simulink model "DAS"  (R2012b)
settings: Solver=FixedStepDiscrete  StartTime=0.0  StopTime=inf  FixedStep=0.1  RelTol=1e-3
PreLoadFcn:
  | if exist('tl_preloadfcn','file'), tl_preloadfcn(gcs,101); end
PostLoadFcn:
  | if exist('tl_postloadfcn','file'), tl_postloadfcn(gcs,101); end
InitFcn:
  | if exist('tlds_init','file'), tlds_init(gcs); end
StartFcn:
  | if exist('tlds_start','file'), tlds_start(gcs); end
StopFcn:
  | if exist('tlds_stop','file'), tlds_stop(gcs); end
undefined symbols (not defined in the file): A, B, C, Dd, DEMO_FAS_Accusti_Threshold_Time, DEMO_FAS_BrakeBooster_Threshold, DEMO_FAS_CC_DELTA, DEMO_FAS_CC_Lvl2_Round, DEMO_FAS_CC_Min_Value, DEMO_FAS_Distance_Treshold_Far, DEMO_FAS_Distance_Treshold_Med, DEMO_FAS_Distance_Treshold_Near, DEMO_FAS_Distronic, DEMO_FAS_Emerg_Brake_Force1, DEMO_FAS_Emerg_Brake_Force2, DEMO_FAS_Emerg_Brake_Time1, DEMO_FAS_Emerg_Brake_Time2, DEMO_FAS_EmergencyBrake, DEMO_FAS_FollowToStop, DEMO_FAS_Limiter, DEMO_FAS_Limiter_DELTA, DEMO_FAS_Neg_Max_ms, DEMO_FAS_Opti_Threshold_Time, DEMO_FAS_Repeater, DEMO_FAS_Repeater_Time, DEMO_FAS_Signdetection, DEMO_FAS_Tempomat
(part 6 of 11)

== system DAS/DEMO_FAS/DEMO_FAS/Subsystem/DEMO_FAS/DEMO_FAS_Funktion/Limiter/Limiter_Function/Limiter_SetValue ==
  LeverUp_stat : Inport
  LeverDown_stat : Inport  Port=2
  Enable : EnablePort
  Constant1 : Constant  Value=0  mask(TL_Constant){data={'date',735340.38498962962}}
      settings: CopyFcn=if exist('tl_reset_reviewflag') == 2, tl_reset_reviewflag(gcbh); end  DeleteFcn=if exist('delete_tlblock','file')==2,delete_tlblock(gcbh);end  NameChangeFcn=if exist('rename_tlblock','file')==2,rename_tlblock(gcbh);end  OpenFcn=if exist('tl_open_blockdlg','file')==2,tl_open_blockdlg(gcbh);else,open_system(gcbh,'parameter');end
      mask Help: eval(['if exist(''tl_online_help'',''file'') == 2, tl_online_help(''Topic'',''TL_Constant''),else, web([''jar:file:///'',matlabroot,''/help/toolbox/simulink/help.jar!/slref/' lower(get_param(gcbh,'Blocktype')) '.html''], ''-helpbrowser''),end'])
      mask Display: plot([-0.05, 1.05, NaN, -0.05, 1.05],[.01, .01, NaN, .99, .99])
  Constant3 : Constant  Value=0  mask(TL_Constant){data={'date',735340.38498962962}}
      settings: CopyFcn=if exist('tl_reset_reviewflag') == 2, tl_reset_reviewflag(gcbh); end  DeleteFcn=if exist('delete_tlblock','file')==2,delete_tlblock(gcbh);end  NameChangeFcn=if exist('rename_tlblock','file')==2,rename_tlblock(gcbh);end  OpenFcn=if exist('tl_open_blockdlg','file')==2,tl_open_blockdlg(gcbh);else,open_system(gcbh,'parameter');end
      mask Help: eval(['if exist(''tl_online_help'',''file'') == 2, tl_online_help(''Topic'',''TL_Constant''),else, web([''jar:file:///'',matlabroot,''/help/toolbox/simulink/help.jar!/slref/' lower(get_param(gcbh,'Blocktype')) '.html''], ''-helpbrowser''),end'])
      mask Display: plot([-0.05, 1.05, NaN, -0.05, 1.05],[.01, .01, NaN, .99, .99])
  Data Store Read1 : DataStoreRead  Description=|  DataStoreName=DEMO_FAS_V_LimiterSetValue  mask(TL_DataStoreRead){data={'logdata',{'plotchannels',[]},'date',735342.5274069329}}
      | Data Store Read block of dSPACE TargetLink.
      | Use this block to specify inputs from global variables within the production code application.
      settings: DeleteFcn=if exist('delete_tlblock','file')==2,delete_tlblock(gcbh);end  NameChangeFcn=if exist('rename_tlblock','file')==2,rename_tlblock(gcbh);end  OpenFcn=if exist('tl_open_blockdlg','file')==2,tl_open_blockdlg(gcbh);else,open_system(gcbh,'parameter');end
      mask Help: eval(['if exist(''tl_online_help'',''file'') == 2, tl_online_help(''Topic'',''TL_DataStoreRead''),else, web([''jar:file:///'',matlabroot,''/help/toolbox/simulink/help.jar!/slref/' lower(get_param(gcbh,'Blocktype')) '.html''], ''-helpbrowser''),end'])
      mask Display: plot([-0.05, 1.05, NaN, -0.05, 1.05],[.01, .01, NaN, .99, .99])
  RelOp1 : RelationalOperator  Description=|  Operator=>  mask(TL_RelationalOperator){data={'logdata',{'plotchannels',[]},'date',735370.55844204861}}
      | Relational operator block of dSPACE TargetLink.
      | 
      | This block performs a relational operation on its two inputs u1 and u2 and produces output according to the following table.
      | If the result is TRUE, the output is 1; if FALSE, it is 0.
      | 
      | Operator   Output
      |  ==        TRUE if u1 is equal to u2
      |  !=        TRUE if u1 is not equal to u2
      |  <         TRUE if u1 is less than u2
      |  <=        TRUE if u1 is less than or equal to u2
      |  >=        TRUE if u1 is greater than or equal to u2
      |  >         TRUE if u1 is greater than u2
      settings: DeleteFcn=if exist('delete_tlblock','file')==2,delete_tlblock(gcbh);end  NameChangeFcn=if exist('rename_tlblock','file')==2,rename_tlblock(gcbh);end  OpenFcn=if exist('tl_open_blockdlg','file')==2,tl_open_blockdlg(gcbh);else,open_system(gcbh,'parameter');end
      mask Help: eval(['if exist(''tl_online_help'',''file'') == 2, tl_online_help(''Topic'',''TL_RelationalOperator''),else, web([''jar:file:///'',matlabroot,''/help/toolbox/simulink/help.jar!/slref/' lower(get_param(gcbh,'Blocktype')) '.html''], ''-helpbrowser''),end'])
      mask Display: plot([-0.05, 1.05, NaN, -0.05, 1.05],[.01, .01, NaN, .99, .99])
  RelOp3 : RelationalOperator  Description=|  Operator=>  mask(TL_RelationalOperator){data={'logdata',{'plotchannels',[]},'date',735370.55844204861}}
      | Relational operator block of dSPACE TargetLink.
      | 
      | This block performs a relational operation on its two inputs u1 and u2 and produces output according to the following table.
      | If the result is TRUE, the output is 1; if FALSE, it is 0.
      | 
      | Operator   Output
      |  ==        TRUE if u1 is equal to u2
      |  !=        TRUE if u1 is not equal to u2
      |  <         TRUE if u1 is less than u2
      |  <=        TRUE if u1 is less than or equal to u2
      |  >=        TRUE if u1 is greater than or equal to u2
      |  >         TRUE if u1 is greater than u2
      settings: DeleteFcn=if exist('delete_tlblock','file')==2,delete_tlblock(gcbh);end  NameChangeFcn=if exist('rename_tlblock','file')==2,rename_tlblock(gcbh);end  OpenFcn=if exist('tl_open_blockdlg','file')==2,tl_open_blockdlg(gcbh);else,open_system(gcbh,'parameter');end
      mask Help: eval(['if exist(''tl_online_help'',''file'') == 2, tl_online_help(''Topic'',''TL_RelationalOperator''),else, web([''jar:file:///'',matlabroot,''/help/toolbox/simulink/help.jar!/slref/' lower(get_param(gcbh,'Blocktype')) '.html''], ''-helpbrowser''),end'])
      mask Display: plot([-0.05, 1.05, NaN, -0.05, 1.05],[.01, .01, NaN, .99, .99])
  VERSION_INFO : Subsystem  mask(VERSION_INFO_BLOCK){versinfo_data=struct('modname','DEMO_FAS/DEMO_FAS_Funktion/Limiter/Limiter_Function/Limiter_SetValue','version','1.1.1','date','18-Apr-2013','author','YVEDUHR','modtype',3,'variant',0,'remark',{{'~'}},'copyright',['Daimler AG'],'SGMLdescr','','prefix','','pfx_act',0,'ntselect',3,'asize',0), versinfo_string=Model: DEMO_FAS/DEMO_FAS_Funktion/Limiter/Limiter_Function/Limiter_SetValue\nVersion: 1.1.1\nDate: 18-Apr-2013\nAuthor: YVEDUHR\nModule: INTERNAL\n\nAll copyrights by Daimler AG}
      mask prompts: versinfo_data "Mask Parameter 1"; versinfo_string "Mask Parameter 2"
      mask help:
      | This is a Version Info Subsystem (empty)
      | All version Information is stored in Parameter "versinfo_data" and displayed
      settings: OpenFcn=edit_subsys_info('init')
      mask Display: disp(versinfo_string);
  V_LimSetValueMinus : Subsystem  TreatAsAtomicUnit=on
  V_LimSetValuePlus : Subsystem  TreatAsAtomicUnit=on
  wires:
  LeverDown_stat/1 -> RelOp1/1
  LeverUp_stat/1 -> RelOp3/1
  Data Store Read1/1 -> V_LimSetValuePlus/1(V_LimiterSetValue), V_LimSetValueMinus/1(V_LimiterSetValue)  "V_LimiterSetValue"
  RelOp3/1 -> V_LimSetValuePlus/Trigger
  Constant3/1 -> RelOp3/2
  Constant1/1 -> RelOp1/2
  RelOp1/1 -> V_LimSetValueMinus/Trigger

== system DAS/DEMO_FAS/DEMO_FAS/Subsystem/DEMO_FAS/DEMO_FAS_Funktion/Limiter/Limiter_Function/Limiter_StartUpSetValue ==
  Trigger : TriggerPort
  Constant : Constant  Value=300  mask(TL_Constant){data={'date',735343.44782005786}}
      settings: CopyFcn=if exist('tl_reset_reviewflag') == 2, tl_reset_reviewflag(gcbh); end  DeleteFcn=if exist('delete_tlblock','file')==2,delete_tlblock(gcbh);end  NameChangeFcn=if exist('rename_tlblock','file')==2,rename_tlblock(gcbh);end  OpenFcn=if exist('tl_open_blockdlg','file')==2,tl_open_blockdlg(gcbh);else,open_system(gcbh,'parameter');end
      mask Help: eval(['if exist(''tl_online_help'',''file'') == 2, tl_online_help(''Topic'',''TL_Constant''),else, web([''jar:file:///'',matlabroot,''/help/toolbox/simulink/help.jar!/slref/' lower(get_param(gcbh,'Blocktype')) '.html''], ''-helpbrowser''),end'])
      mask Display: plot([-0.05, 1.05, NaN, -0.05, 1.05],[.01, .01, NaN, .99, .99])
  Data Store Write : DataStoreWrite  Description=|  DataStoreName=DEMO_FAS_V_CCSetValue  mask(TL_DataStoreWrite){data={'date',735342.52876391204}}
      | Data Store Write block of dSPACE TargetLink.
      | Use this block to specify outputs to global variables within the production code application.
      settings: DeleteFcn=if exist('delete_tlblock','file')==2,delete_tlblock(gcbh);end  NameChangeFcn=if exist('rename_tlblock','file')==2,rename_tlblock(gcbh);end  OpenFcn=if exist('tl_open_blockdlg','file')==2,tl_open_blockdlg(gcbh);else,open_system(gcbh,'parameter');end
      mask Help: eval(['if exist(''tl_online_help'',''file'') == 2, tl_online_help(''Topic'',''TL_DataStoreWrite''),else, web([''jar:file:///'',matlabroot,''/help/toolbox/simulink/help.jar!/slref/' lower(get_param(gcbh,'Blocktype')) '.html''], ''-helpbrowser''),end'])
      mask Display: plot([-0.05, 1.05, NaN, -0.05, 1.05],[.01, .01, NaN, .99, .99])
  VERSION_INFO : Subsystem  mask(VERSION_INFO_BLOCK){versinfo_data=struct('modname','DEMO_FAS/DEMO_FAS_Funktion/Limiter/Limiter_Function/Limiter_StartUpSetValue','version','1.1.1','date','18-Apr-2013','author','YVEDUHR','modtype',3,'variant',0,'remark',{{'~'}},'copyright',['Daimler AG'],'SGMLdescr','','prefix','','pfx_act',0,'ntselect',3,'asize',0), versinfo_string=Model: DEMO_FAS/DEMO_FAS_Funktion/Limiter/Limiter_Function/Limiter_StartUpSetValue\nVersion: 1.1.1\nDate: 18-Apr-2013\nAuthor: YVEDUHR\nModule: INTERNAL\n\nAll copyrights by Daimler AG}
      mask prompts: versinfo_data "Mask Parameter 1"; versinfo_string "Mask Parameter 2"
      mask help:
      | This is a Version Info Subsystem (empty)
      | All version Information is stored in Parameter "versinfo_data" and displayed
      settings: OpenFcn=edit_subsys_info('init')
      mask Display: disp(versinfo_string);
  wires:
  Constant/1 -> Data Store Write/1

== system DAS/DEMO_FAS/DEMO_FAS/Subsystem/DEMO_FAS/DEMO_FAS_Funktion/Limiter/Limiter_Function/SysInit ==
  Memory_Init : UnitDelay  Description=|  InitialCondition=1  SampleTime=dT  mask(TL_UnitDelay){data={'logdata',{'plotchannels',[]},'output',{'type','Bool'},'state',{'type','Bool'},'date',734383.73415}}
      | Unit Delay block of dSPACE TargetLink.
      | 
      | Output signal is equal to the input signal of the last sample step:
      | 
      |         y(k) = u(k-1).
      | 
      | In the 1st sampling step, the output signal is initialized with 'initial condition':
      | 
      |         y(0) = initial condition
      settings: CopyFcn=if exist('tl_reset_reviewflag') == 2, tl_reset_reviewflag(gcbh); end  DeleteFcn=if exist('delete_tlblock','file')==2,delete_tlblock(gcbh);end  NameChangeFcn=if exist('rename_tlblock','file')==2,rename_tlblock(gcbh);end  OpenFcn=if exist('tl_open_blockdlg','file')==2,tl_open_blockdlg(gcbh);else,open_system(gcbh,'parameter');end
      mask Help: eval(['if exist(''tl_online_help'',''file'') == 2, tl_online_help(''Topic'',''TL_UnitDelay''),else, web([''jar:file:///'',matlabroot,''/help/toolbox/simulink/help.jar!/slref/' lower(get_param(gcbh,'Blocktype')) '.html''], ''-helpbrowser''),end'])
      mask Display: plot([-0.05, 1.05, NaN, -0.05, 1.05],[.01, .01, NaN, .99, .99])
  Zero_Init : Constant  Description=|  Value=0  SampleTime=dT  mask(TL_Constant){data={'date',734383.73414928245}}
      | Constant block of dSPACE TargetLink.
      | 
      | Output signal keeps the given constant value.
      settings: DeleteFcn=if exist('delete_tlblock','file')==2,delete_tlblock(gcbh);end  NameChangeFcn=if exist('rename_tlblock','file')==2,rename_tlblock(gcbh);end  OpenFcn=if exist('tl_open_blockdlg','file')==2,tl_open_blockdlg(gcbh);else,open_system(gcbh,'parameter');end
      mask Help: eval(['if exist(''tl_online_help'',''file'') == 2, tl_online_help(''Topic'',''TL_Constant''),else, web([''jar:file:///'',matlabroot,''/help/toolbox/simulink/help.jar!/slref/' lower(get_param(gcbh,'Blocktype')) '.html''], ''-helpbrowser''),end'])
      mask Display: plot([-0.05, 1.05, NaN, -0.05, 1.05],[.01, .01, NaN, .99, .99])
  y : Outport
  wires:
  Zero_Init/1 -> Memory_Init/1
  Memory_Init/1 -> y/1

== system DAS/DEMO_FAS/DEMO_FAS/Subsystem/DEMO_FAS/DEMO_FAS_Funktion/Limiter/Limiter_Function/VERSION_INFO ==
  Copyright : Subsystem
      mask help: Copyright
      mask Display: disp('All copyrights by DaimlerChrysler');

== system DAS/DEMO_FAS/DEMO_FAS/Subsystem/DEMO_FAS/DEMO_FAS_Funktion/Limiter/VERSION_INFO/Copyright ==

== system DAS/DEMO_FAS/DEMO_FAS/Subsystem/DEMO_FAS/DEMO_FAS_Funktion/Tempomat/Tempomat_Function/CC_Enabled ==
  CC_active_b : Inport
  V_Vehicle_kmh : Inport  Port=2
  Bus Creator : BusCreator  Inputs=1
  Bus Creator1 : BusCreator  Inputs=1
  Bus Selector : BusSelector  OutputSignals=V_CC_delta_kmh
  If : If  IfExpression=u1
  Merge : Merge  Description=|  mask(TL_Merge){data={'date',735441.37248614582}}
      | Merge block of dSPACE TargetLink.
      | 
      | Use this block instead of Simulink's Merge block if you wish to control how merge variables should be generated.
      settings: CopyFcn=if exist('tl_reset_reviewflag') == 2, tl_reset_reviewflag(gcbh); end  DeleteFcn=if exist('delete_tlblock','file')==2,delete_tlblock(gcbh);end  NameChangeFcn=if exist('rename_tlblock','file')==2,rename_tlblock(gcbh);end  OpenFcn=if exist('tl_open_blockdlg','file')==2,tl_open_blockdlg(gcbh);else,open_system(gcbh,'parameter');end
      mask Help: eval(['if exist(''tl_online_help'',''file'') == 2, tl_online_help(''Topic'',''TL_Merge''),else, web([''jar:file:///'',matlabroot,''/help/toolbox/simulink/help.jar!/slref/' lower(get_param(gcbh,'Blocktype')) '.html''], ''-helpbrowser''),end'])
      mask Display: plot([-0.05, 1.05, NaN, -0.05, 1.05],[.01, .01, NaN, .99, .99])
  Tempomat_Active : Subsystem  TreatAsAtomicUnit=on
  Tempomat_Deactive : Subsystem  TreatAsAtomicUnit=on
  VERSION_INFO : Subsystem  mask(VERSION_INFO_BLOCK){versinfo_data=struct('modname','DEMO_FAS/DEMO_FAS_Funktion/Tempomat/Tempomat_Function/CC_Enabled','version','1.1.1','date','18-Apr-2013','author','YVEDUHR','modtype',3,'variant',0,'remark',{{'~'}},'copyright',['Daimler AG'],'SGMLdescr','','prefix','','pfx_act',0,'ntselect',3,'asize',0), versinfo_string=Model: DEMO_FAS/DEMO_FAS_Funktion/Tempomat/Tempomat_Function/CC_Enabled\nVersion: 1.1.1\nDate: 18-Apr-2013\nAuthor: YVEDUHR\nModule: INTERNAL\n\nAll copyrights by Daimler AG}
      mask prompts: versinfo_data "Mask Parameter 1"; versinfo_string "Mask Parameter 2"
      mask help:
      | This is a Version Info Subsystem (empty)
      | All version Information is stored in Parameter "versinfo_data" and displayed
      settings: OpenFcn=edit_subsys_info('init')
      mask Display: disp(versinfo_string);
  V_CC_delta_kmh : Outport  InitialOutput=0
  wires:
  If/1 -> Tempomat_Active/Action
  V_Vehicle_kmh/1 -> Tempomat_Active/1(V_Vehicle_kmh)
  Tempomat_Active/1(V_CC_delta_kmh) -> Bus Creator/1
  Bus Creator/1 -> Merge/1
  Tempomat_Deactive/1(V_CC_delta_kmh) -> Bus Creator1/1
  Bus Creator1/1 -> Merge/2
  Merge/1 -> Bus Selector/1  "V_CC_delta_kmh"
  Bus Selector/1 -> V_CC_delta_kmh/1  "<V_CC_delta_kmh>"
  CC_active_b/1 -> If/1
  If/2 -> Tempomat_Deactive/Action

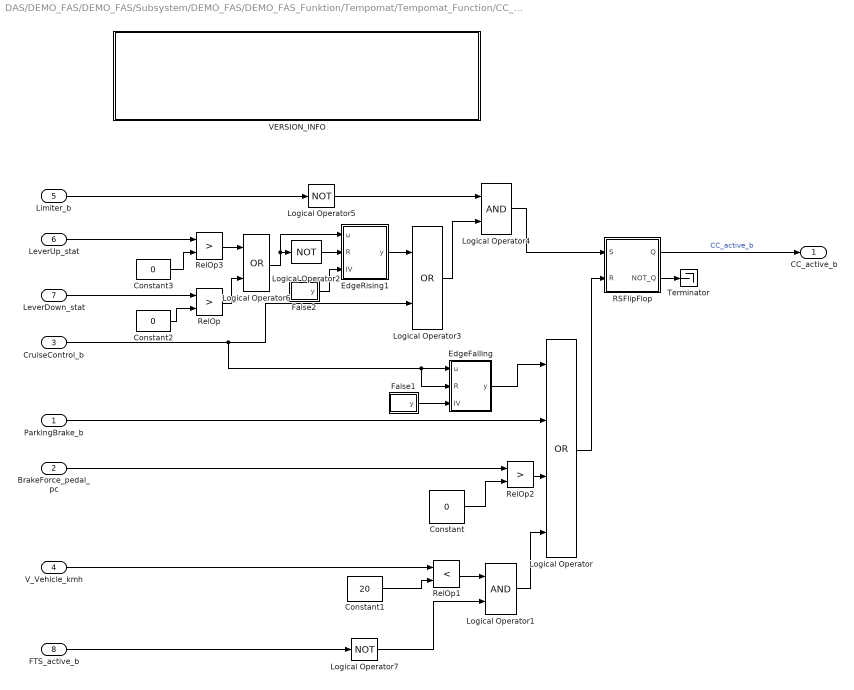
== system DAS/DEMO_FAS/DEMO_FAS/Subsystem/DEMO_FAS/DEMO_FAS_Funktion/Tempomat/Tempomat_Function/CC_On_Off ==
  ParkingBrake_b : Inport
  BrakeForce_pedal_pc : Inport  Port=2
  CruiseControl_b : Inport  Port=3
  V_Vehicle_kmh : Inport  Port=4
  Limiter_b : Inport  Port=5
  LeverUp_stat : Inport  Port=6
  LeverDown_stat : Inport  Port=7
  FTS_active_b : Inport  Port=8
  Constant : Constant  Value=0  mask(TL_Constant){data={'date',735340.38498962962}}
      settings: CopyFcn=if exist('tl_reset_reviewflag') == 2, tl_reset_reviewflag(gcbh); end  DeleteFcn=if exist('delete_tlblock','file')==2,delete_tlblock(gcbh);end  NameChangeFcn=if exist('rename_tlblock','file')==2,rename_tlblock(gcbh);end  OpenFcn=if exist('tl_open_blockdlg','file')==2,tl_open_blockdlg(gcbh);else,open_system(gcbh,'parameter');end
      mask Help: eval(['if exist(''tl_online_help'',''file'') == 2, tl_online_help(''Topic'',''TL_Constant''),else, web([''jar:file:///'',matlabroot,''/help/toolbox/simulink/help.jar!/slref/' lower(get_param(gcbh,'Blocktype')) '.html''], ''-helpbrowser''),end'])
      mask Display: plot([-0.05, 1.05, NaN, -0.05, 1.05],[.01, .01, NaN, .99, .99])
  Constant1 : Constant  Value=20  mask(TL_Constant){data={'date',735343.57031072921}}
      settings: CopyFcn=if exist('tl_reset_reviewflag') == 2, tl_reset_reviewflag(gcbh); end  DeleteFcn=if exist('delete_tlblock','file')==2,delete_tlblock(gcbh);end  NameChangeFcn=if exist('rename_tlblock','file')==2,rename_tlblock(gcbh);end  OpenFcn=if exist('tl_open_blockdlg','file')==2,tl_open_blockdlg(gcbh);else,open_system(gcbh,'parameter');end
      mask Help: eval(['if exist(''tl_online_help'',''file'') == 2, tl_online_help(''Topic'',''TL_Constant''),else, web([''jar:file:///'',matlabroot,''/help/toolbox/simulink/help.jar!/slref/' lower(get_param(gcbh,'Blocktype')) '.html''], ''-helpbrowser''),end'])
      mask Display: plot([-0.05, 1.05, NaN, -0.05, 1.05],[.01, .01, NaN, .99, .99])
  Constant2 : Constant  Value=0  mask(TL_Constant){data={'date',735340.38498962962}}
      settings: CopyFcn=if exist('tl_reset_reviewflag') == 2, tl_reset_reviewflag(gcbh); end  DeleteFcn=if exist('delete_tlblock','file')==2,delete_tlblock(gcbh);end  NameChangeFcn=if exist('rename_tlblock','file')==2,rename_tlblock(gcbh);end  OpenFcn=if exist('tl_open_blockdlg','file')==2,tl_open_blockdlg(gcbh);else,open_system(gcbh,'parameter');end
      mask Help: eval(['if exist(''tl_online_help'',''file'') == 2, tl_online_help(''Topic'',''TL_Constant''),else, web([''jar:file:///'',matlabroot,''/help/toolbox/simulink/help.jar!/slref/' lower(get_param(gcbh,'Blocktype')) '.html''], ''-helpbrowser''),end'])
      mask Display: plot([-0.05, 1.05, NaN, -0.05, 1.05],[.01, .01, NaN, .99, .99])
  Constant3 : Constant  Value=0  mask(TL_Constant){data={'date',735340.38498962962}}
      settings: CopyFcn=if exist('tl_reset_reviewflag') == 2, tl_reset_reviewflag(gcbh); end  DeleteFcn=if exist('delete_tlblock','file')==2,delete_tlblock(gcbh);end  NameChangeFcn=if exist('rename_tlblock','file')==2,rename_tlblock(gcbh);end  OpenFcn=if exist('tl_open_blockdlg','file')==2,tl_open_blockdlg(gcbh);else,open_system(gcbh,'parameter');end
      mask Help: eval(['if exist(''tl_online_help'',''file'') == 2, tl_online_help(''Topic'',''TL_Constant''),else, web([''jar:file:///'',matlabroot,''/help/toolbox/simulink/help.jar!/slref/' lower(get_param(gcbh,'Blocktype')) '.html''], ''-helpbrowser''),end'])
      mask Display: plot([-0.05, 1.05, NaN, -0.05, 1.05],[.01, .01, NaN, .99, .99])
  EdgeFalling : Subsystem  mask(TLMSR_V200_EdgeFalling){dT=-1, YName=}
      mask prompts: dT "Sample Time"; YName "Y OutName"
      mask help:
      | The output indicates TRUE if the input value changes from TRUE to FALSE.
      | Reset input 'R' on TRUE will write the initial value 'IV' to the internal memory.
      mask init:
      | % TL block lines
      | x1=[0 0 1 1 0];
      | y1=[1 0 0 1 1];
      | x2=[1 0];
      | y2=[.96 .96];
      | x3=[0 1];
      | y3=[.04 .04];
      | 
      | tl_act_sg_init_blk;
      mask Help:
      | <HTML>
      | <HEAD>
      | <META HTTP-EQUIV="Content-Type" CONTENT="text/html; charset=iso-8859-1">
      | <TITLE>Help</TITLE>
      | </HEAD>
      | <BODY>
      | 
      | <B><FONT FACE="Arial"><P>Function:</P>
      | </B><P>The block detects a falling edge of the logical input signal <FONT FACE="Courier New">u</FONT> and indicates this change at the output <FONT FACE="Courier New">y</FONT> for one cycle.</P>
      | 
      | <B><P>In-/Outputs:</P>
      | </B>
      | <P><U>Input</U></P>
      | <P>The block input </FONT><FONT FACE="Courier New">u</FONT><FONT FACE="Arial"> must be connected to the input signal.</P>
      | 
      | <U><P>Reset / Initial Value</P>
      | </U><P>If the reset input </FONT><FONT FACE="Courier New">R</FONT><FONT FACE="Arial"> gets a '1' signal the block will write the initial value <FONT FACE="Courier New">IV</FONT> to its internal memory. A logical '0' at <FONT FACE="Courier New">IV</FONT>
      | will prevent the output to become TRUE during reset.</P>
      | 
      | <U><P>Output</P>
      | </U><P>The output </FONT><FONT FACE="Courier New">y</FONT><FONT FACE="Arial"> shows '1' if a falling edge at the input signal <FONT FACE="Courier New">u</FONT> is detected.</P>
      | </FONT></BODY>
      | </HTML>
      mask Display:
      | plot(x1,y1,x2,y2,x3,y3);
      | image(imread('EdgeFalling.tif','tif'),[0.25,0.2,0.5,0.6])
  EdgeRising1 : Subsystem  mask(TLMSR_V200_EdgeRising){dT=-1, YName=}
      mask prompts: dT "Sampe Time"; YName "Y OutName"
      mask help:
      | The output indicates TRUE if the input value changes from FALSE to TRUE.
      | Reset input 'R' on TRUE will write the initial value 'IV' to the internal memory.
      mask init:
      | % TL block lines
      | x1=[0 0 1 1 0];
      | y1=[1 0 0 1 1];
      | x2=[1 0];
      | y2=[.96 .96];
      | x3=[0 1];
      | y3=[.04 .04];
      | 
      | tl_act_sg_init_blk;
      mask Help:
      | <HTML>
      | <HEAD>
      | <META HTTP-EQUIV="Content-Type" CONTENT="text/html; charset=iso-8859-1">
      | <TITLE>Help</TITLE>
      | </HEAD>
      | <BODY>
      | 
      | <B><FONT FACE="Arial"><P>Function:</P>
      | </B><P>The block detects a rising edge of the logical input signal <FONT FACE="Courier New">u</FONT> and indicates this change at the output <FONT FACE="Courier New">y</FONT> for one cycle.</P>
      | 
      | <B><P>In-/Outputs:</P>
      | </B>
      | <P><U>Input</U></P>
      | <P>The block input </FONT><FONT FACE="Courier New">u</FONT><FONT FACE="Arial"> must be connected to the input signal.</P>
      | 
      | <U><P>Reset / Initial Value</P>
      | </U><P>If the reset input </FONT><FONT FACE="Courier New">R</FONT><FONT FACE="Arial"> gets a '1' signal the block will write the initial value <FONT FACE="Courier New">IV</FONT> to its internal memory. A logical '1' at <FONT FACE="Courier New">IV</FONT>
      | will prevent the output to become TRUE during reset.</P>
      | 
      | <U><P>Output</P>
      | </U><P>The output </FONT><FONT FACE="Courier New">y</FONT><FONT FACE="Arial"> shows '1' if a rising edge at the input signal <FONT FACE="Courier New">u</FONT> is detected.</P>
      | </FONT></BODY>
      | </HTML>
      mask Display:
      | plot(x1,y1,x2,y2,x3,y3);
      | image(imread('EdgeRising.tif','tif'),[0.25,0.2,0.5,0.6])
  False1 : Subsystem  mask(TLACT_SG_V200_False){}
      mask help: False
      mask init:
      | % TL block lines
      | x1=[0 0 1 1 0];
      | y1=[1 0 0 1 1];
      | x2=[1 0];
      | y2=[.9 .9];
      | x3=[0 1];
      | y3=[.1 .1];
      settings: OpenFcn=open_system([gcb, '/Zero'], 'OpenFcn')
      mask Display:
      | plot(x1,y1,x2,y2,x3,y3);
      | disp('False');
  False2 : Subsystem  mask(TLACT_SG_V200_False){}
      mask help: False
      mask init:
      | % TL block lines
      | x1=[0 0 1 1 0];
      | y1=[1 0 0 1 1];
      | x2=[1 0];
      | y2=[.9 .9];
      | x3=[0 1];
      | y3=[.1 .1];
      settings: OpenFcn=open_system([gcb, '/Zero'], 'OpenFcn')
      mask Display:
      | plot(x1,y1,x2,y2,x3,y3);
      | disp('False');
  Logical Operator : Logic  Operator=OR  Inputs=4  AllPortsSameDT=off  OutDataTypeStr=boolean  mask(TL_LogicalOperator){data={'date',735343.59622336808}}
      settings: DeleteFcn=if exist('delete_tlblock','file')==2,delete_tlblock(gcbh);end  NameChangeFcn=if exist('rename_tlblock','file')==2,rename_tlblock(gcbh);end  OpenFcn=if exist('tl_open_blockdlg','file')==2,tl_open_blockdlg(gcbh);else,open_system(gcbh,'parameter');end
      mask Help: eval(['if exist(''tl_online_help'',''file'') == 2, tl_online_help(''Topic'',''TL_LogicalOperator''),else, web([''jar:file:///'',matlabroot,''/help/toolbox/simulink/help.jar!/slref/' lower(get_param(gcbh,'Blocktype')) '.html''], ''-helpbrowser''),end'])
      mask Display: plot([-0.05, 1.05, NaN, -0.05, 1.05],[.01, .01, NaN, .99, .99])
  Logical Operator1 : Logic  AllPortsSameDT=off  OutDataTypeStr=boolean  mask(TL_LogicalOperator){data={'date',735346.45212662034}}
      settings: DeleteFcn=if exist('delete_tlblock','file')==2,delete_tlblock(gcbh);end  NameChangeFcn=if exist('rename_tlblock','file')==2,rename_tlblock(gcbh);end  OpenFcn=if exist('tl_open_blockdlg','file')==2,tl_open_blockdlg(gcbh);else,open_system(gcbh,'parameter');end
      mask Help: eval(['if exist(''tl_online_help'',''file'') == 2, tl_online_help(''Topic'',''TL_LogicalOperator''),else, web([''jar:file:///'',matlabroot,''/help/toolbox/simulink/help.jar!/slref/' lower(get_param(gcbh,'Blocktype')) '.html''], ''-helpbrowser''),end'])
      mask Display: plot([-0.05, 1.05, NaN, -0.05, 1.05],[.01, .01, NaN, .99, .99])
  Logical Operator2 : Logic  Operator=NOT  Inputs=1  AllPortsSameDT=off  OutDataTypeStr=boolean  mask(TL_LogicalOperator){data={'date',735339.71002042829}}
      settings: DeleteFcn=if exist('delete_tlblock','file')==2,delete_tlblock(gcbh);end  NameChangeFcn=if exist('rename_tlblock','file')==2,rename_tlblock(gcbh);end  OpenFcn=if exist('tl_open_blockdlg','file')==2,tl_open_blockdlg(gcbh);else,open_system(gcbh,'parameter');end
      mask Help: eval(['if exist(''tl_online_help'',''file'') == 2, tl_online_help(''Topic'',''TL_LogicalOperator''),else, web([''jar:file:///'',matlabroot,''/help/toolbox/simulink/help.jar!/slref/' lower(get_param(gcbh,'Blocktype')) '.html''], ''-helpbrowser''),end'])
      mask Display: plot([-0.05, 1.05, NaN, -0.05, 1.05],[.01, .01, NaN, .99, .99])
  Logical Operator3 : Logic  Operator=OR  AllPortsSameDT=off  OutDataTypeStr=boolean  mask(TL_LogicalOperator){data={'date',735375.57476618059}}
      settings: DeleteFcn=if exist('delete_tlblock','file')==2,delete_tlblock(gcbh);end  NameChangeFcn=if exist('rename_tlblock','file')==2,rename_tlblock(gcbh);end  OpenFcn=if exist('tl_open_blockdlg','file')==2,tl_open_blockdlg(gcbh);else,open_system(gcbh,'parameter');end
      mask Help: eval(['if exist(''tl_online_help'',''file'') == 2, tl_online_help(''Topic'',''TL_LogicalOperator''),else, web([''jar:file:///'',matlabroot,''/help/toolbox/simulink/help.jar!/slref/' lower(get_param(gcbh,'Blocktype')) '.html''], ''-helpbrowser''),end'])
      mask Display: plot([-0.05, 1.05, NaN, -0.05, 1.05],[.01, .01, NaN, .99, .99])
  Logical Operator4 : Logic  AllPortsSameDT=off  OutDataTypeStr=boolean  mask(TL_LogicalOperator){data={'date',735346.45212662034}}
      settings: DeleteFcn=if exist('delete_tlblock','file')==2,delete_tlblock(gcbh);end  NameChangeFcn=if exist('rename_tlblock','file')==2,rename_tlblock(gcbh);end  OpenFcn=if exist('tl_open_blockdlg','file')==2,tl_open_blockdlg(gcbh);else,open_system(gcbh,'parameter');end
      mask Help: eval(['if exist(''tl_online_help'',''file'') == 2, tl_online_help(''Topic'',''TL_LogicalOperator''),else, web([''jar:file:///'',matlabroot,''/help/toolbox/simulink/help.jar!/slref/' lower(get_param(gcbh,'Blocktype')) '.html''], ''-helpbrowser''),end'])
      mask Display: plot([-0.05, 1.05, NaN, -0.05, 1.05],[.01, .01, NaN, .99, .99])
  Logical Operator5 : Logic  Operator=NOT  Inputs=1  AllPortsSameDT=off  OutDataTypeStr=boolean  mask(TL_LogicalOperator){data={'date',735346.45245848375}}
      settings: DeleteFcn=if exist('delete_tlblock','file')==2,delete_tlblock(gcbh);end  NameChangeFcn=if exist('rename_tlblock','file')==2,rename_tlblock(gcbh);end  OpenFcn=if exist('tl_open_blockdlg','file')==2,tl_open_blockdlg(gcbh);else,open_system(gcbh,'parameter');end
      mask Help: eval(['if exist(''tl_online_help'',''file'') == 2, tl_online_help(''Topic'',''TL_LogicalOperator''),else, web([''jar:file:///'',matlabroot,''/help/toolbox/simulink/help.jar!/slref/' lower(get_param(gcbh,'Blocktype')) '.html''], ''-helpbrowser''),end'])
      mask Display: plot([-0.05, 1.05, NaN, -0.05, 1.05],[.01, .01, NaN, .99, .99])
  Logical Operator6 : Logic  Operator=OR  AllPortsSameDT=off  OutDataTypeStr=boolean  mask(TL_LogicalOperator){data={'date',735375.57446980325}}
      settings: DeleteFcn=if exist('delete_tlblock','file')==2,delete_tlblock(gcbh);end  NameChangeFcn=if exist('rename_tlblock','file')==2,rename_tlblock(gcbh);end  OpenFcn=if exist('tl_open_blockdlg','file')==2,tl_open_blockdlg(gcbh);else,open_system(gcbh,'parameter');end
      mask Help: eval(['if exist(''tl_online_help'',''file'') == 2, tl_online_help(''Topic'',''TL_LogicalOperator''),else, web([''jar:file:///'',matlabroot,''/help/toolbox/simulink/help.jar!/slref/' lower(get_param(gcbh,'Blocktype')) '.html''], ''-helpbrowser''),end'])
      mask Display: plot([-0.05, 1.05, NaN, -0.05, 1.05],[.01, .01, NaN, .99, .99])
  Logical Operator7 : Logic  Operator=NOT  Inputs=1  AllPortsSameDT=off  OutDataTypeStr=boolean  mask(TL_LogicalOperator){data={'date',735346.45245848375}}
      settings: DeleteFcn=if exist('delete_tlblock','file')==2,delete_tlblock(gcbh);end  NameChangeFcn=if exist('rename_tlblock','file')==2,rename_tlblock(gcbh);end  OpenFcn=if exist('tl_open_blockdlg','file')==2,tl_open_blockdlg(gcbh);else,open_system(gcbh,'parameter');end
      mask Help: eval(['if exist(''tl_online_help'',''file'') == 2, tl_online_help(''Topic'',''TL_LogicalOperator''),else, web([''jar:file:///'',matlabroot,''/help/toolbox/simulink/help.jar!/slref/' lower(get_param(gcbh,'Blocktype')) '.html''], ''-helpbrowser''),end'])
      mask Display: plot([-0.05, 1.05, NaN, -0.05, 1.05],[.01, .01, NaN, .99, .99])
  RSFlipFlop : Subsystem  mask(TLMSR_V200_RSFlipFlop){dT=-1, QName=, QNName=}
      mask prompts: dT "SampleTime"; QName "Q OutName"; QNName "QN OutName"
      mask help: A flip flop. The 'R' input (reset) dominates the 'S' input (set).
      mask init:
      | % TL block lines
      | x1=[0 0 1 1 0];
      | y1=[1 0 0 1 1];
      | x2=[1 0];
      | y2=[.96 .96];
      | x3=[0 1];
      | y3=[.04 .04];
      | 
      | tl_act_sg_init_blk;
      mask Help:
      | <HTML>
      | <HEAD>
      | <META HTTP-EQUIV="Content-Type" CONTENT="text/html; charset=iso-8859-1">
      | <TITLE>test</TITLE>
      | </HEAD>
      | 
      | <B><FONT FACE="Arial"><P>Function:</P>
      | </B><P>The block provides the function of a RS-Flip-Flop with the reset input </FONT><FONT FACE="Courier New">R</FONT><FONT FACE="Arial"> dominating over the set input </FONT><FONT FACE="Courier New">S</FONT><FONT FACE="Arial">. An inverted output </FONT><FONT FACE="Courier New">/Q</FONT><FONT FACE="Arial"> is provided.</P>
      | </FONT>
      | <TABLE BORDER CELLSPACING=1 CELLPADDING=4 WIDTH=506>
      | <TR><TD WIDTH="25%" VALIGN="TOP">
      | <B><FONT FACE="Arial"><P ALIGN="CENTER">S</B></FONT></TD>
      | <TD WIDTH="25%" VALIGN="TOP">
      | <B><FONT FACE="Arial"><P ALIGN="CENTER">R</B></FONT></TD>
      | <TD WIDTH="25%" VALIGN="TOP">
      | <B><FONT FACE="Arial"><P ALIGN="CENTER">Q</B></FONT></TD>
      | <TD WIDTH="25%" VALIGN="TOP">
      | <B><FONT FACE="Arial"><P ALIGN="CENTER">/Q</B></FONT></TD>
      | </TR>
      | <TR><TD WIDTH="25%" VALIGN="TOP">
      | <FONT FACE="Arial"><P ALIGN="CENTER">0</FONT></TD>
      | <TD WIDTH="25%" VALIGN="TOP">
      | <FONT FACE="Arial"><P ALIGN="CENTER">0</FONT></TD>
      | <TD WIDTH="25%" VALIGN="TOP">
      | <FONT FACE="Arial"><P ALIGN="CENTER">Q(n-1)</FONT></TD>
      | <TD WIDTH="25%" VALIGN="TOP">
      | <FONT FACE="Arial"><P ALIGN="CENTER">/Q(n-1)</FONT></TD>
      | </TR>
      | <TR><TD WIDTH="25%" VALIGN="TOP">
      | <FONT FACE="Arial"><P ALIGN="CENTER">0</FONT></TD>
      | <TD WIDTH="25%" VALIGN="TOP">
      | <FONT FACE="Arial"><P ALIGN="CENTER">1</FONT></TD>
      | <TD WIDTH="25%" VALIGN="TOP">
      | <FONT FACE="Arial"><P ALIGN="CENTER">0</FONT></TD>
      | <TD WIDTH="25%" VALIGN="TOP">
      | <FONT FACE="Arial"><P ALIGN="CENTER">1</FONT></TD>
      | </TR>
      | <TR><TD WIDTH="25%" VALIGN="TOP">
      | <FONT FACE="Arial"><P ALIGN="CENTER">1</FONT></TD>
      | <TD WIDTH="25%" VALIGN="TOP">
      | <FONT FACE="Arial"><P ALIGN="CENTER">0</FONT></TD>
      | <TD WIDTH="25%" VALIGN="TOP">
      | <FONT FACE="Arial"><P ALIGN="CENTER">1</FONT></TD>
      | <TD WIDTH="25%" VALIGN="TOP">
      | <FONT FACE="Arial"><P ALIGN="CENTER">0</FONT></TD>
      | </TR>
      | <TR><TD WIDTH="25%" VALIGN="TOP">
      | <FONT FACE="Arial"><P ALIGN="CENTER">1</FONT></TD>
      | <TD WIDTH="25%" VALIGN="TOP">
      | <FONT FACE="Arial"><P ALIGN="CENTER">1</FONT></TD>
      | <TD WIDTH="25%" VALIGN="TOP">
      | <FONT FACE="Arial"><P ALIGN="CENTER">0</FONT></TD>
      | <TD WIDTH="25%" VALIGN="TOP">
      | <FONT FACE="Arial"><P ALIGN="CENTER">1</FONT></TD>
      | </TR>
      | </TABLE>
      | 
      | <FONT FACE="Arial">
      | <B><P>In-/Outputs:</P>
      | </B><U><P>S</P>
      | </U><P>The set input </FONT><FONT FACE="Courier New">S</FONT><FONT FACE="Arial"> on '1' will set the output </FONT><FONT FACE="Courier New">Q</FONT><FONT FACE="Arial"> if the reset input </FONT><FONT FACE="Courier New">R</FONT><FONT FACE="Arial"> is '0'.</P>
      | <U><P>R</P>
      | </U><P>The reset input </FONT><FONT FACE="Courier New">R</FONT><FONT FACE="Arial"> on '1' will reset the output </FONT><FONT FACE="Courier New">Q</FONT><FONT FACE="Arial">.</P>
      | <U><P>Q, /Q</P>
      | </U><P>The output </FONT><FONT FACE="Courier New">Q</FONT><FONT FACE="Arial"> shows the state of the internal memory. </FONT><FONT FACE="Courier New">/Q</FONT><FONT FACE="Arial"> contains the inverted state of </FONT><FONT FACE="Courier New">Q</FONT><FONT FACE="Arial">.</P></FONT>
      | </HTML>
      mask Display:
      | plot(x1,y1,x2,y2,x3,y3);
      | image(imread('RSFlipFlop.tif','tif'),[0.05,0.1,0.9,0.8])
  RelOp : RelationalOperator  Description=|  Operator=>  mask(TL_RelationalOperator){data={'logdata',{'plotchannels',[]},'date',735370.55844204861}}
      | Relational operator block of dSPACE TargetLink.
      | 
      | This block performs a relational operation on its two inputs u1 and u2 and produces output according to the following table.
      | If the result is TRUE, the output is 1; if FALSE, it is 0.
      | 
      | Operator   Output
      |  ==        TRUE if u1 is equal to u2
      |  !=        TRUE if u1 is not equal to u2
      |  <         TRUE if u1 is less than u2
      |  <=        TRUE if u1 is less than or equal to u2
      |  >=        TRUE if u1 is greater than or equal to u2
      |  >         TRUE if u1 is greater than u2
      settings: DeleteFcn=if exist('delete_tlblock','file')==2,delete_tlblock(gcbh);end  NameChangeFcn=if exist('rename_tlblock','file')==2,rename_tlblock(gcbh);end  OpenFcn=if exist('tl_open_blockdlg','file')==2,tl_open_blockdlg(gcbh);else,open_system(gcbh,'parameter');end
      mask Help: eval(['if exist(''tl_online_help'',''file'') == 2, tl_online_help(''Topic'',''TL_RelationalOperator''),else, web([''jar:file:///'',matlabroot,''/help/toolbox/simulink/help.jar!/slref/' lower(get_param(gcbh,'Blocktype')) '.html''], ''-helpbrowser''),end'])
      mask Display: plot([-0.05, 1.05, NaN, -0.05, 1.05],[.01, .01, NaN, .99, .99])
  RelOp1 : RelationalOperator  Description=|  Operator=<  mask(TL_RelationalOperator){data={'logdata',{'plotchannels',[]},'date',735343.59715890046}}
      | Relational operator block of dSPACE TargetLink.
      | 
      | This block performs a relational operation on its two inputs u1 and u2 and produces output according to the following table.
      | If the result is TRUE, the output is 1; if FALSE, it is 0.
      | 
      | Operator   Output
      |  ==        TRUE if u1 is equal to u2
      |  !=        TRUE if u1 is not equal to u2
      |  <         TRUE if u1 is less than u2
      |  <=        TRUE if u1 is less than or equal to u2
      |  >=        TRUE if u1 is greater than or equal to u2
      |  >         TRUE if u1 is greater than u2
      settings: DeleteFcn=if exist('delete_tlblock','file')==2,delete_tlblock(gcbh);end  NameChangeFcn=if exist('rename_tlblock','file')==2,rename_tlblock(gcbh);end  OpenFcn=if exist('tl_open_blockdlg','file')==2,tl_open_blockdlg(gcbh);else,open_system(gcbh,'parameter');end
      mask Help: eval(['if exist(''tl_online_help'',''file'') == 2, tl_online_help(''Topic'',''TL_RelationalOperator''),else, web([''jar:file:///'',matlabroot,''/help/toolbox/simulink/help.jar!/slref/' lower(get_param(gcbh,'Blocktype')) '.html''], ''-helpbrowser''),end'])
      mask Display: plot([-0.05, 1.05, NaN, -0.05, 1.05],[.01, .01, NaN, .99, .99])
  RelOp2 : RelationalOperator  Description=|  Operator=>  mask(TL_RelationalOperator){data={'logdata',{'plotchannels',[]},'date',735354.41198150464}}
      | Relational operator block of dSPACE TargetLink.
      | 
      | This block performs a relational operation on its two inputs u1 and u2 and produces output according to the following table.
      | If the result is TRUE, the output is 1; if FALSE, it is 0.
      | 
      | Operator   Output
      |  ==        TRUE if u1 is equal to u2
      |  !=        TRUE if u1 is not equal to u2
      |  <         TRUE if u1 is less than u2
      |  <=        TRUE if u1 is less than or equal to u2
      |  >=        TRUE if u1 is greater than or equal to u2
      |  >         TRUE if u1 is greater than u2
      settings: DeleteFcn=if exist('delete_tlblock','file')==2,delete_tlblock(gcbh);end  NameChangeFcn=if exist('rename_tlblock','file')==2,rename_tlblock(gcbh);end  OpenFcn=if exist('tl_open_blockdlg','file')==2,tl_open_blockdlg(gcbh);else,open_system(gcbh,'parameter');end
      mask Help: eval(['if exist(''tl_online_help'',''file'') == 2, tl_online_help(''Topic'',''TL_RelationalOperator''),else, web([''jar:file:///'',matlabroot,''/help/toolbox/simulink/help.jar!/slref/' lower(get_param(gcbh,'Blocktype')) '.html''], ''-helpbrowser''),end'])
      mask Display: plot([-0.05, 1.05, NaN, -0.05, 1.05],[.01, .01, NaN, .99, .99])
  RelOp3 : RelationalOperator  Description=|  Operator=>  mask(TL_RelationalOperator){data={'logdata',{'plotchannels',[]},'date',735370.55844204861}}
      | Relational operator block of dSPACE TargetLink.
      | 
      | This block performs a relational operation on its two inputs u1 and u2 and produces output according to the following table.
      | If the result is TRUE, the output is 1; if FALSE, it is 0.
      | 
      | Operator   Output
      |  ==        TRUE if u1 is equal to u2
      |  !=        TRUE if u1 is not equal to u2
      |  <         TRUE if u1 is less than u2
      |  <=        TRUE if u1 is less than or equal to u2
      |  >=        TRUE if u1 is greater than or equal to u2
      |  >         TRUE if u1 is greater than u2
      settings: DeleteFcn=if exist('delete_tlblock','file')==2,delete_tlblock(gcbh);end  NameChangeFcn=if exist('rename_tlblock','file')==2,rename_tlblock(gcbh);end  OpenFcn=if exist('tl_open_blockdlg','file')==2,tl_open_blockdlg(gcbh);else,open_system(gcbh,'parameter');end
      mask Help: eval(['if exist(''tl_online_help'',''file'') == 2, tl_online_help(''Topic'',''TL_RelationalOperator''),else, web([''jar:file:///'',matlabroot,''/help/toolbox/simulink/help.jar!/slref/' lower(get_param(gcbh,'Blocktype')) '.html''], ''-helpbrowser''),end'])
      mask Display: plot([-0.05, 1.05, NaN, -0.05, 1.05],[.01, .01, NaN, .99, .99])
  Terminator : Terminator
  VERSION_INFO : Subsystem  mask(VERSION_INFO_BLOCK){versinfo_data=struct('modname','DEMO_FAS/DEMO_FAS_Funktion/Tempomat/Tempomat_Function/CC_On_Off','version','1.1.1','date','19-Apr-2013','author','YVEDUHR','modtype',3,'variant',0,'remark',{{'~'}},'copyright',['Daimler AG'],'SGMLdescr','','prefix','','pfx_act',0,'ntselect',3,'asize',0), versinfo_string=Model: DEMO_FAS/DEMO_FAS_Funktion/Tempomat/Tempomat_Function/CC_On_Off\nVersion: 1.1.1\nDate: 19-Apr-2013\nAuthor: YVEDUHR\nModule: INTERNAL\n\nAll copyrights by Daimler AG}
      mask prompts: versinfo_data "Mask Parameter 1"; versinfo_string "Mask Parameter 2"
      mask help:
      | This is a Version Info Subsystem (empty)
      | All version Information is stored in Parameter "versinfo_data" and displayed
      settings: OpenFcn=edit_subsys_info('init')
      mask Display: disp(versinfo_string);
  CC_active_b : Outport
  wires:
  Logical Operator4/1 -> RSFlipFlop/1(S)
  Logical Operator/1 -> RSFlipFlop/2(R)
  RelOp2/1 -> Logical Operator/3
  Constant/1 -> RelOp2/2
  ParkingBrake_b/1 -> Logical Operator/2
  RSFlipFlop/2(NOT_Q) -> Terminator/1
  BrakeForce_pedal_pc/1 -> RelOp2/1
  Constant1/1 -> RelOp1/2
  RSFlipFlop/1(Q) -> CC_active_b/1  "CC_active_b"
  RelOp1/1 -> Logical Operator1/1
  LeverDown_stat/1 -> RelOp/1
  LeverUp_stat/1 -> RelOp3/1
  V_Vehicle_kmh/1 -> RelOp1/1
  EdgeFalling/1(y) -> Logical Operator/1
  False1/1(y) -> EdgeFalling/3(IV)
  CruiseControl_b/1 -> Logical Operator3/2, EdgeFalling/1(u), EdgeFalling/2(R)
  Limiter_b/1 -> Logical Operator5/1
  Logical Operator5/1 -> Logical Operator4/1
  RelOp3/1 -> Logical Operator6/1
  RelOp/1 -> Logical Operator6/2
  Constant2/1 -> RelOp/2
  Constant3/1 -> RelOp3/2
  Logical Operator3/1 -> Logical Operator4/2
  Logical Operator2/1 -> EdgeRising1/2(R)
  False2/1(y) -> EdgeRising1/3(IV)
  Logical Operator6/1 -> Logical Operator2/1, EdgeRising1/1(u)
  EdgeRising1/1(y) -> Logical Operator3/1
  Logical Operator1/1 -> Logical Operator/4
  Logical Operator7/1 -> Logical Operator1/2
  FTS_active_b/1 -> Logical Operator7/1
